simulink model "exer"  (R2020b)
settings: Solver=VariableStepAuto  StartTime=0.0  StopTime=30.0  RelTol=1e-3
undefined symbols (not defined in the file or in its folder): A_kalman, L
settings Model: Creator=renato  LastModifiedBy=renato

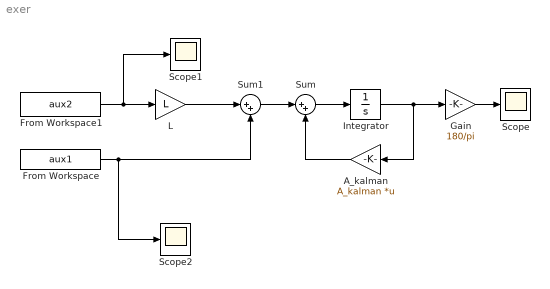
== system exer ==
  A_kalman : Gain  Gain=A_kalman  Multiplication=Matrix(K*u)
  From Workspace : FromWorkspace  VariableName=aux1
  From Workspace1 : FromWorkspace  VariableName=aux2
  Gain : Gain  Gain=180/pi
  Integrator : Integrator
  L : Gain  Gain=L
  Scope : Scope
  Scope1 : Scope
  Scope2 : Scope
  Sum : Sum  Inputs=|++
  Sum1 : Sum  Inputs=|++
  wires:
  From Workspace1/1 -> Scope1/1, L/1
  From Workspace/1 -> Scope2/1, Sum1/2
  A_kalman/1 -> Sum/2
  Sum1/1 -> Sum/1
  Sum/1 -> Integrator/1
  Integrator/1 -> Gain/1, A_kalman/1
  L/1 -> Sum1/1
  Gain/1 -> Scope/1
